simulink model "programa"  (Simulink 8.2)
settings: Solver=FixedStepDiscrete  SolverMode=SingleTasking  StartTime=0.0  StopTime=inf  FixedStep=0.001  RelTol=1e-3
PreLoadFcn:
  | waijung.modelPreload; % Required for working with Waijung Blockset. Do not remove.
undefined symbols (not defined in the file): ARM, Link, LQFP144, MDK, ST, STM32F405ZG
libraries: stm32f4_adc_lib x3, stm32f4_device_config_lib x1, USBVCP_STM32F4 x1
CloseFcn:
  | waijung.modelClose; % Required for working with Waijung Blockset. Do not remove.
settings Model: Creator=Sr Antonio  LastModifiedBy=gonza
settings OptimizationCC: OptimizeModelRefInitCode=on  LifeSpan=1
settings DebuggingCC: FcnCallInpInsideContextMsg=EnableAllAsWarning
settings HardwareCC: ProdEndianess=LittleEndian  ProdHWDeviceType=ARM Compatible->Cortex - M4  TargetEndianess=LittleEndian  TargetHWDeviceType=ARM Compatible->Cortex - M4
settings RTWCC: SystemTargetFile=stm32f4.tlc  GenerateMakefile=off  TemplateMakefile=ert_default_tmf  Description=STM32F4 Target  ProcessScript=stm32f4_make_rtw_hook
settings CodeAppCC: IgnoreCustomStorageClasses=off  CustomSymbolStrType=$N$R$M  InternalIdentifier=Classic
settings STFCustomTargetCC: CodeReplacementLibrary=ANSI_C  ModelReferenceCompliant=off  CombineOutputUpdateFcns=on  ERTCustomFileBanners=on  SupportContinuousTime=off  SupportNonInlinedSFcns=off  MATLABClassNameForMDSCustomization=Simulink.SoftwareTarget.ERTCustomization  GRTInterface=off  SystemTargetFile=stm32f4.tlc
settings ERTTargetCC: CodeReplacementLibrary=ANSI_C  MultiwordLength=2048  ModelReferenceCompliant=off  ParMdlRefBuildCompliant=off  CompOptLevelCompliant=off  ConcurrentExecutionCompliant=off  ERTFirstTimeCompliant=off  ModelStepFunctionPrototypeControlCompliant=off  CPPClassGenCompliant=off  ExtModeMexFile=noextcomm  InlinedParameterPlacement=NonHierarchical  ERTSrcFileBannerTemplate=stm32f4_code_template.cgt  ERTHdrFileBannerTemplate=stm32f4_code_template.cgt  ERTDataSrcFileTemplate=stm32f4_code_template.cgt  ERTDataHdrFileTemplate=stm32f4_code_template.cgt  ERTCustomFileTemplate=stm32f4_file_process.tlc  ConvertIfToSwitch=off  SuppressUnreachableDefaultCases=off

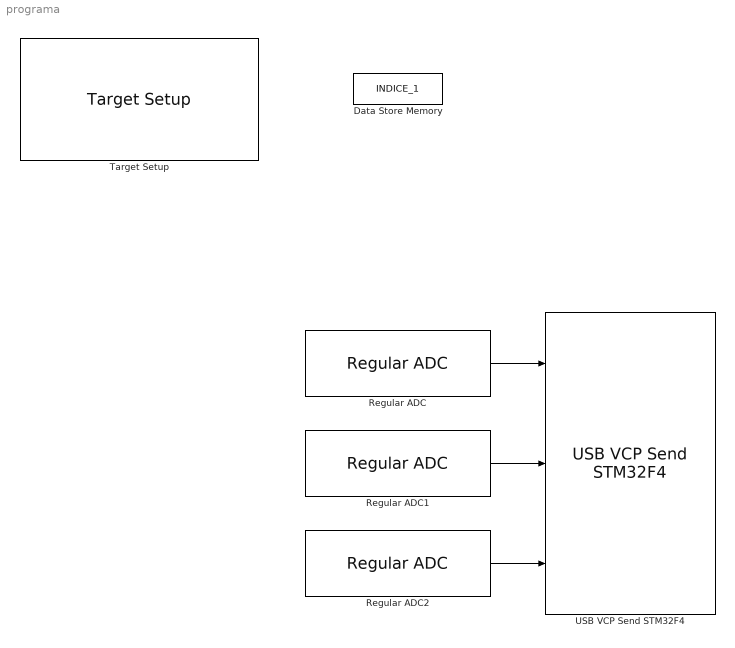
== system programa ==
  Data Store Memory : DataStoreMemory  DataStoreName=INDICE_1  ReadBeforeWriteMsg=warning  WriteAfterWriteMsg=warning  WriteAfterReadMsg=warning  OutDataTypeStr=uint16
  Regular ADC : stm32f4_adc_lib/Regular ADC  adcmodule=1  outputdatatype=Single  prescaler=8  prescalerstr=ADC_Prescaler_Div8  chsamplingtime=Auto  chsamplingtimestr=ADC_SampleTime_480Cycles  read_an0=on  read_an1=off  read_an2=off  read_an3=off  read_an4=off  read_an5=off  read_an6=off  read_an7=off  read_an8=off  read_an9=off  read_an10=off  read_an11=off  read_an12=off  read_an13=off  read_an14=off  read_an15=off  read_an16=off  read_an17=off  read_an18=off  pinstr=GPIO_Pin_0  usedpinarray="[1  0  0  0  0  0  0  0  0  0  0  0  0  0  0  0  0  0  0]"  usedportidarray=[0]  usedpinidarray=[0]  usedpinidcount=1  sampletime=0.001  blockid=RegularADC  enablecustomportlabel=off  cinputportlabel=0  coutputportlabel=Out1, Out2
  Regular ADC1 : stm32f4_adc_lib/Regular ADC  adcmodule=2  outputdatatype=Single  prescaler=8  prescalerstr=ADC_Prescaler_Div8  chsamplingtime=Auto  chsamplingtimestr=ADC_SampleTime_480Cycles  read_an0=off  read_an1=on  read_an2=off  read_an3=off  read_an4=off  read_an5=off  read_an6=off  read_an7=off  read_an8=off  read_an9=off  read_an10=off  read_an11=off  read_an12=off  read_an13=off  read_an14=off  read_an15=off  read_an16=off  read_an17=off  read_an18=off  pinstr=GPIO_Pin_0  usedpinarray="[1  0  0  0  0  0  0  0  0  0  0  0  0  0  0  0  0  0  0]"  usedportidarray=[0]  usedpinidarray=[0]  usedpinidcount=1  sampletime=0.001  blockid=RegularADC1  enablecustomportlabel=off  cinputportlabel=0  coutputportlabel=Out1, Out2
  Regular ADC2 : stm32f4_adc_lib/Regular ADC  adcmodule=3  outputdatatype=Single  prescaler=8  prescalerstr=ADC_Prescaler_Div8  chsamplingtime=Auto  chsamplingtimestr=ADC_SampleTime_480Cycles  read_an0=off  read_an1=off  read_an2=on  read_an3=off  read_an4=off  read_an5=off  read_an6=off  read_an7=off  read_an8=off  read_an9=off  read_an10=off  read_an11=off  read_an12=off  read_an13=off  read_an14=off  read_an15=off  read_an16=off  read_an17=off  read_an18=off  pinstr=GPIO_Pin_0  usedpinarray="[1  0  0  0  0  0  0  0  0  0  0  0  0  0  0  0  0  0  0]"  usedportidarray=[0]  usedpinidarray=[0]  usedpinidcount=1  sampletime=0.001  blockid=RegularADC2  enablecustomportlabel=off  cinputportlabel=0  coutputportlabel=Out1, Out2
  Target Setup : stm32f4_device_config_lib/Target Setup  Priority=100  compiler=MDK-ARM  previous_compiler=MDK-ARM  mcu=STM32F405ZG (LQFP144)  mcustr=STM32F405ZG  clockconfig=STM32F4DISCOVERY Default (HSEOSC-8MHz/HCLK-168MHz)  system_stm32f4xx_c_path=C:\BC_3\targets\stm32f4_target\stm32f4\utils\STM32F4xx_AN3988_V1.0.1\stm32f4_default\hseosc8mhz  showmemoryconfiguration=on  stacksize=0x2000  heapsize=0x2000  enableautocompiledownload=on  fullchiperase=off  programmerinterface=ST-Link  editctrlstr=on  compilercontrolstr=-c --cpu Cortex-M4.fp -g -O3 --apcs=interwork --split_sections $(INCLUDES)  assemblercontrolstr="--cpu Cortex-M4.fp -g --apcs=interwork  --xref $(INCLUDES)"  linkercontrolstr="--cpu Cortex-M4.fp --strict --scatter \"$(MODELNAME).sct\" --summary_stderr --info summarysizes --map --xref --callgraph --symbols --info sizes --info totals --info unused --info veneers  --list \".\\$(MODELNAME).map\" -o $(MODELNAME).axf"  runafterdownload=on  execprofile=None  profileruart=1  profilerbaud=115200  profilertxpin=Not used  profilerinitstr=0.001,168000000,168000,115200,0  manualsetsampletime=on  sampletime=0.001  blockid=TargetSetup  systickreloadvalue=168000  hseval=8000000  lastprofileruart=1  hclk=168000000  flashorigin=0x08000000  flashlength=0x00100000  ramorigin=0x20000000  ramlength=0x00020000  useextram=off
  USB VCP Send STM32F4 : USBVCP_STM32F4/USB VCP Send STM32F4  speed="USB 1.1   12Mbit/s"  data_size=2048 Bytes  header_data='0E 0E'  binary_data='single single single'  terminator_data='0A 0A'  sampletime=0.001
  wires:
  Regular ADC/1 -> USB VCP Send STM32F4/1
  Regular ADC1/1 -> USB VCP Send STM32F4/2
  Regular ADC2/1 -> USB VCP Send STM32F4/3
